simulink model "IEEE34_SPSload"  (R2021b)
settings: Solver=ode4  StartTime=0.0  StopTime=5  FixedStep=50e-6  RelTol=1e-3
PreLoadFcn:
  | pGain = 0.05; % Gain of random perturbation (pu)
  | pGainAP = 0.01; % Gain of sinusoidal active power variation (pu)
  | pGainRP = 0.01; % Gain of sinusoidal reactive power variation (pu)
  | pFreqAP = 0.03; % Frequency of sinusoidal active power variation (Hz)
  | pFreqRP = 0.03; % Frequency of sinusoidal reactive power variation (Hz)
  | 
  | init_IEEE34nodetestfeeder;
InitFcn:
  | pGain = 0.05; % Gain of random perturbation (pu)
  | pGainAP = 0.01; % Gain of sinusoidal active power variation (pu)
  | pGainRP = 0.01; % Gain of sinusoidal reactive power variation (pu)
  | pFreqAP = 0.03; % Frequency of sinusoidal active power variation (Hz)
  | pFreqRP = 0.03; % Frequency of sinusoidal reactive power variation (Hz)
  | 
  | init_IEEE34nodetestfeeder;
values from neighbouring files (symbols this model uses):
  fNom = f    (= 60)    [init_IEEE34nodetestfeeder.m]
  loadcoeff = 1.0    (= 1)    [init_IEEE34nodetestfeeder.m]
  Ts = 50e-6    (= 5e-05)    [init_IEEE34nodetestfeeder.m]
  vNomMV = VsubL    (= 24900)    [init_IEEE34nodetestfeeder.m]
  VsubL = 24.9e3    (= 24900)    [init_IEEE34nodetestfeeder.m]
  VxfmL = 4.16e3    (= 4160)    [init_IEEE34nodetestfeeder.m]
undefined symbols (not defined in the file or in its folder): Ac, Bc, Cc, Dc, find_system, j
libraries: spsSeriesRLCBranchLib x418, spsGroundLib x242, simulink_extras x176, spsVoltageMeasurementLib x106, spsRMSLib x96, spsControlledCurrentSourceLib x94, spsThreePhaseVIMeasurementLib x37, spsMutualInductanceLib x24, spsCurrentMeasurementLib x12, spsOnDelayLib x12, spsLinearTransformerLib x6, spsControlledVoltageSourceLib x6
(part 14 of 33)

== system IEEE34_SPSload/SM_IEEE34/DL_844-1/Load B2/model ==
  v : Inport
  PQ : Inport  Port=2
  Break Alg. Loop : Subsystem
  Complex to Magnitude-Angle : ComplexToMagnitudeAngle
  Complex to Real-Imag1 : ComplexToRealImag
  Constant : Constant
  Demux : Demux  Outputs=2
      settings: DisplayOption=none
  Divide : Product  Inputs=**
  IC1 : InitialCondition
  IC2 : InitialCondition
  Magnitude-Angle to Complex : MagnitudeAngleToComplex
  PLL : Subsystem  mask{freq=fnom}
      mask prompts: freq "Initial frequency (Hz)"
  Positive Sequence current : Subsystem
  RMS1 : spsRMSLib/RMS  TrueRMS=on  Freq=fnom  RMSInit=1  Ts=0
  Real-Imag to Complex : RealImagToComplex
  Real-Imag to Complex1 : RealImagToComplex
  Sum : Sum
  Trigonometric Function1 : Trigonometry
  V> pu : Gain  Gain=1/Vbase/sqrt(3)  SaturateOnIntegerOverflow=on  OutDataTypeStr=Inherit: Same as input  ParamDataTypeStr=Inherit: Same as input
  V> pu1 : Gain  Gain=sqrt(2)  SaturateOnIntegerOverflow=on  OutDataTypeStr=Inherit: Same as input  ParamDataTypeStr=Inherit: Same as input
  i : Outport  VectorParamsAs1DForOutWhenUnconnected=off
  m : Outport  Port=2  VectorParamsAs1DForOutWhenUnconnected=off
  wires:
  V> pu/1 -> PLL/1(v (pu)), V> pu1/1
  Real-Imag to Complex/1 -> Positive Sequence current/1(V1(pu))
  Positive Sequence current/1(I1(A)) -> Break Alg. Loop/1(In)
  PQ/1 -> Demux/1
  Demux/1 -> Real-Imag to Complex1/1
  Demux/2 -> Real-Imag to Complex1/2
  Real-Imag to Complex1/1 -> Positive Sequence current/2(S_ext)
  Positive Sequence current/2(VPQ) -> m/1
  v/1 -> IC2/1
  Complex to Real-Imag1/1 -> Real-Imag to Complex/1
  Complex to Real-Imag1/2 -> Real-Imag to Complex/2
  Magnitude-Angle to Complex/1 -> Complex to Real-Imag1/1
  Constant/1 -> PLL/2(freq (pu))
  PLL/1(alpha (rad)) -> Magnitude-Angle to Complex/2
  Complex to Magnitude-Angle/2 -> Sum/2
  PLL/2(wt) -> Sum/1
  Sum/1 -> Trigonometric Function1/1
  Trigonometric Function1/1 -> Divide/2
  Complex to Magnitude-Angle/1 -> Divide/1
  Divide/1 -> i/1
  Break Alg. Loop/1(Out) -> Complex to Magnitude-Angle/1
  RMS1/1 -> IC1/1
  IC1/1 -> Magnitude-Angle to Complex/1
  V> pu1/1 -> RMS1/1
  IC2/1 -> V> pu/1

== system IEEE34_SPSload/SM_IEEE34/DL_844-846/Load B/Measurement list ==
  In1 : Inport
  Bus Creator1 : BusCreator  Inputs=3
  Demux : Demux  Outputs=[1,1,1]
  Out1 : Outport  VectorParamsAs1DForOutWhenUnconnected=off
  wires:
  Demux/3 -> Bus Creator1/3  "Reactive power Q (var)"
  Demux/1 -> Bus Creator1/1  "Positive-sequence voltage V (pu)"
  Demux/2 -> Bus Creator1/2  "Active power P (W)"
  Bus Creator1/1 -> Out1/1
  In1/1 -> Demux/1

== system IEEE34_SPSload/SM_IEEE34/DL_844-846/Load B/model ==
  v : Inport
  PQ : Inport  Port=2
  Break Alg. Loop : Subsystem
  Complex to Magnitude-Angle : ComplexToMagnitudeAngle
  Complex to Real-Imag1 : ComplexToRealImag
  Constant : Constant
  Demux : Demux  Outputs=2
      settings: DisplayOption=none
  Divide : Product  Inputs=**
  IC1 : InitialCondition
  IC2 : InitialCondition
  Magnitude-Angle to Complex : MagnitudeAngleToComplex
  PLL : Subsystem  mask{freq=fnom}
      mask prompts: freq "Initial frequency (Hz)"
  Positive Sequence current : Subsystem
  RMS1 : spsRMSLib/RMS  TrueRMS=on  Freq=fnom  RMSInit=1  Ts=0
  Real-Imag to Complex : RealImagToComplex
  Real-Imag to Complex1 : RealImagToComplex
  Sum : Sum
  Trigonometric Function1 : Trigonometry
  V> pu : Gain  Gain=1/Vbase/sqrt(3)  SaturateOnIntegerOverflow=on  OutDataTypeStr=Inherit: Same as input  ParamDataTypeStr=Inherit: Same as input
  V> pu1 : Gain  Gain=sqrt(2)  SaturateOnIntegerOverflow=on  OutDataTypeStr=Inherit: Same as input  ParamDataTypeStr=Inherit: Same as input
  i : Outport  VectorParamsAs1DForOutWhenUnconnected=off
  m : Outport  Port=2  VectorParamsAs1DForOutWhenUnconnected=off
  wires:
  V> pu/1 -> PLL/1(v (pu)), V> pu1/1
  Real-Imag to Complex/1 -> Positive Sequence current/1(V1(pu))
  Positive Sequence current/1(I1(A)) -> Break Alg. Loop/1(In)
  PQ/1 -> Demux/1
  Demux/1 -> Real-Imag to Complex1/1
  Demux/2 -> Real-Imag to Complex1/2
  Real-Imag to Complex1/1 -> Positive Sequence current/2(S_ext)
  Positive Sequence current/2(VPQ) -> m/1
  v/1 -> IC2/1
  Complex to Real-Imag1/1 -> Real-Imag to Complex/1
  Complex to Real-Imag1/2 -> Real-Imag to Complex/2
  Magnitude-Angle to Complex/1 -> Complex to Real-Imag1/1
  Constant/1 -> PLL/2(freq (pu))
  PLL/1(alpha (rad)) -> Magnitude-Angle to Complex/2
  Complex to Magnitude-Angle/2 -> Sum/2
  PLL/2(wt) -> Sum/1
  Sum/1 -> Trigonometric Function1/1
  Trigonometric Function1/1 -> Divide/2
  Complex to Magnitude-Angle/1 -> Divide/1
  Divide/1 -> i/1
  Break Alg. Loop/1(Out) -> Complex to Magnitude-Angle/1
  RMS1/1 -> IC1/1
  IC1/1 -> Magnitude-Angle to Complex/1
  V> pu1/1 -> RMS1/1
  IC2/1 -> V> pu/1

== system IEEE34_SPSload/SM_IEEE34/DL_844-846/Load B1/Measurement list ==
  In1 : Inport
  Bus Creator1 : BusCreator  Inputs=3
  Demux : Demux  Outputs=[1,1,1]
  Out1 : Outport  VectorParamsAs1DForOutWhenUnconnected=off
  wires:
  Demux/3 -> Bus Creator1/3  "Reactive power Q (var)"
  Demux/1 -> Bus Creator1/1  "Positive-sequence voltage V (pu)"
  Demux/2 -> Bus Creator1/2  "Active power P (W)"
  Bus Creator1/1 -> Out1/1
  In1/1 -> Demux/1

== system IEEE34_SPSload/SM_IEEE34/DL_844-846/Load B1/model ==
  v : Inport
  PQ : Inport  Port=2
  Break Alg. Loop : Subsystem
  Complex to Magnitude-Angle : ComplexToMagnitudeAngle
  Complex to Real-Imag1 : ComplexToRealImag
  Constant : Constant
  Demux : Demux  Outputs=2
      settings: DisplayOption=none
  Divide : Product  Inputs=**
  IC1 : InitialCondition
  IC2 : InitialCondition
  Magnitude-Angle to Complex : MagnitudeAngleToComplex
  PLL : Subsystem  mask{freq=fnom}
      mask prompts: freq "Initial frequency (Hz)"
  Positive Sequence current : Subsystem
  RMS1 : spsRMSLib/RMS  TrueRMS=on  Freq=fnom  RMSInit=1  Ts=0
  Real-Imag to Complex : RealImagToComplex
  Real-Imag to Complex1 : RealImagToComplex
  Sum : Sum
  Trigonometric Function1 : Trigonometry
  V> pu : Gain  Gain=1/Vbase/sqrt(3)  SaturateOnIntegerOverflow=on  OutDataTypeStr=Inherit: Same as input  ParamDataTypeStr=Inherit: Same as input
  V> pu1 : Gain  Gain=sqrt(2)  SaturateOnIntegerOverflow=on  OutDataTypeStr=Inherit: Same as input  ParamDataTypeStr=Inherit: Same as input
  i : Outport  VectorParamsAs1DForOutWhenUnconnected=off
  m : Outport  Port=2  VectorParamsAs1DForOutWhenUnconnected=off
  wires:
  V> pu/1 -> PLL/1(v (pu)), V> pu1/1
  Real-Imag to Complex/1 -> Positive Sequence current/1(V1(pu))
  Positive Sequence current/1(I1(A)) -> Break Alg. Loop/1(In)
  PQ/1 -> Demux/1
  Demux/1 -> Real-Imag to Complex1/1
  Demux/2 -> Real-Imag to Complex1/2
  Real-Imag to Complex1/1 -> Positive Sequence current/2(S_ext)
  Positive Sequence current/2(VPQ) -> m/1
  v/1 -> IC2/1
  Complex to Real-Imag1/1 -> Real-Imag to Complex/1
  Complex to Real-Imag1/2 -> Real-Imag to Complex/2
  Magnitude-Angle to Complex/1 -> Complex to Real-Imag1/1
  Constant/1 -> PLL/2(freq (pu))
  PLL/1(alpha (rad)) -> Magnitude-Angle to Complex/2
  Complex to Magnitude-Angle/2 -> Sum/2
  PLL/2(wt) -> Sum/1
  Sum/1 -> Trigonometric Function1/1
  Trigonometric Function1/1 -> Divide/2
  Complex to Magnitude-Angle/1 -> Divide/1
  Divide/1 -> i/1
  Break Alg. Loop/1(Out) -> Complex to Magnitude-Angle/1
  RMS1/1 -> IC1/1
  IC1/1 -> Magnitude-Angle to Complex/1
  V> pu1/1 -> RMS1/1
  IC2/1 -> V> pu/1

== system IEEE34_SPSload/SM_IEEE34/DL_844-846/Load B2/Measurement list ==
  In1 : Inport
  Bus Creator1 : BusCreator  Inputs=3
  Demux : Demux  Outputs=[1,1,1]
  Out1 : Outport  VectorParamsAs1DForOutWhenUnconnected=off
  wires:
  In1/1 -> Demux/1
  Bus Creator1/1 -> Out1/1
  Demux/2 -> Bus Creator1/2  "Active power P (W)"
  Demux/1 -> Bus Creator1/1  "Positive-sequence voltage V (pu)"
  Demux/3 -> Bus Creator1/3  "Reactive power Q (var)"

== system IEEE34_SPSload/SM_IEEE34/DL_844-846/Load B2/model ==
  v : Inport
  PQ : Inport  Port=2
  Break Alg. Loop : Subsystem
  Complex to Magnitude-Angle : ComplexToMagnitudeAngle
  Complex to Real-Imag1 : ComplexToRealImag
  Constant : Constant
  Demux : Demux  Outputs=2
      settings: DisplayOption=none
  Divide : Product  Inputs=**
  IC1 : InitialCondition
  IC2 : InitialCondition
  Magnitude-Angle to Complex : MagnitudeAngleToComplex
  PLL : Subsystem  mask{freq=fnom}
      mask prompts: freq "Initial frequency (Hz)"
  Positive Sequence current : Subsystem
  RMS1 : spsRMSLib/RMS  TrueRMS=on  Freq=fnom  RMSInit=1  Ts=0
  Real-Imag to Complex : RealImagToComplex
  Real-Imag to Complex1 : RealImagToComplex
  Sum : Sum
  Trigonometric Function1 : Trigonometry
  V> pu : Gain  Gain=1/Vbase/sqrt(3)  SaturateOnIntegerOverflow=on  OutDataTypeStr=Inherit: Same as input  ParamDataTypeStr=Inherit: Same as input
  V> pu1 : Gain  Gain=sqrt(2)  SaturateOnIntegerOverflow=on  OutDataTypeStr=Inherit: Same as input  ParamDataTypeStr=Inherit: Same as input
  i : Outport  VectorParamsAs1DForOutWhenUnconnected=off
  m : Outport  Port=2  VectorParamsAs1DForOutWhenUnconnected=off
  wires:
  IC2/1 -> V> pu/1
  V> pu1/1 -> RMS1/1
  IC1/1 -> Magnitude-Angle to Complex/1
  RMS1/1 -> IC1/1
  Break Alg. Loop/1(Out) -> Complex to Magnitude-Angle/1
  Divide/1 -> i/1
  Complex to Magnitude-Angle/1 -> Divide/1
  Trigonometric Function1/1 -> Divide/2
  Sum/1 -> Trigonometric Function1/1
  PLL/2(wt) -> Sum/1
  Complex to Magnitude-Angle/2 -> Sum/2
  PLL/1(alpha (rad)) -> Magnitude-Angle to Complex/2
  Constant/1 -> PLL/2(freq (pu))
  Magnitude-Angle to Complex/1 -> Complex to Real-Imag1/1
  Complex to Real-Imag1/2 -> Real-Imag to Complex/2
  Complex to Real-Imag1/1 -> Real-Imag to Complex/1
  v/1 -> IC2/1
  Positive Sequence current/2(VPQ) -> m/1
  Real-Imag to Complex1/1 -> Positive Sequence current/2(S_ext)
  Demux/2 -> Real-Imag to Complex1/2
  Demux/1 -> Real-Imag to Complex1/1
  PQ/1 -> Demux/1
  Positive Sequence current/1(I1(A)) -> Break Alg. Loop/1(In)
  Real-Imag to Complex/1 -> Positive Sequence current/1(V1(pu))
  V> pu/1 -> V> pu1/1, PLL/1(v (pu))

== system IEEE34_SPSload/SM_IEEE34/DL_846-1/Load B/Measurement list ==
  In1 : Inport
  Bus Creator1 : BusCreator  Inputs=3
  Demux : Demux  Outputs=[1,1,1]
  Out1 : Outport  VectorParamsAs1DForOutWhenUnconnected=off
  wires:
  In1/1 -> Demux/1
  Bus Creator1/1 -> Out1/1
  Demux/2 -> Bus Creator1/2  "Active power P (W)"
  Demux/1 -> Bus Creator1/1  "Positive-sequence voltage V (pu)"
  Demux/3 -> Bus Creator1/3  "Reactive power Q (var)"

== system IEEE34_SPSload/SM_IEEE34/DL_846-1/Load B/model ==
  v : Inport
  PQ : Inport  Port=2
  Break Alg. Loop : Subsystem
  Complex to Magnitude-Angle : ComplexToMagnitudeAngle
  Complex to Real-Imag1 : ComplexToRealImag
  Constant : Constant
  Demux : Demux  Outputs=2
      settings: DisplayOption=none
  Divide : Product  Inputs=**
  IC1 : InitialCondition
  IC2 : InitialCondition
  Magnitude-Angle to Complex : MagnitudeAngleToComplex
  PLL : Subsystem  mask{freq=fnom}
      mask prompts: freq "Initial frequency (Hz)"
  Positive Sequence current : Subsystem
  RMS1 : spsRMSLib/RMS  TrueRMS=on  Freq=fnom  RMSInit=1  Ts=0
  Real-Imag to Complex : RealImagToComplex
  Real-Imag to Complex1 : RealImagToComplex
  Sum : Sum
  Trigonometric Function1 : Trigonometry
  V> pu : Gain  Gain=1/Vbase/sqrt(3)  SaturateOnIntegerOverflow=on  OutDataTypeStr=Inherit: Same as input  ParamDataTypeStr=Inherit: Same as input
  V> pu1 : Gain  Gain=sqrt(2)  SaturateOnIntegerOverflow=on  OutDataTypeStr=Inherit: Same as input  ParamDataTypeStr=Inherit: Same as input
  i : Outport  VectorParamsAs1DForOutWhenUnconnected=off
  m : Outport  Port=2  VectorParamsAs1DForOutWhenUnconnected=off
  wires:
  IC2/1 -> V> pu/1
  V> pu1/1 -> RMS1/1
  IC1/1 -> Magnitude-Angle to Complex/1
  RMS1/1 -> IC1/1
  Break Alg. Loop/1(Out) -> Complex to Magnitude-Angle/1
  Divide/1 -> i/1
  Complex to Magnitude-Angle/1 -> Divide/1
  Trigonometric Function1/1 -> Divide/2
  Sum/1 -> Trigonometric Function1/1
  PLL/2(wt) -> Sum/1
  Complex to Magnitude-Angle/2 -> Sum/2
  PLL/1(alpha (rad)) -> Magnitude-Angle to Complex/2
  Constant/1 -> PLL/2(freq (pu))
  Magnitude-Angle to Complex/1 -> Complex to Real-Imag1/1
  Complex to Real-Imag1/2 -> Real-Imag to Complex/2
  Complex to Real-Imag1/1 -> Real-Imag to Complex/1
  v/1 -> IC2/1
  Positive Sequence current/2(VPQ) -> m/1
  Real-Imag to Complex1/1 -> Positive Sequence current/2(S_ext)
  Demux/2 -> Real-Imag to Complex1/2
  Demux/1 -> Real-Imag to Complex1/1
  PQ/1 -> Demux/1
  Positive Sequence current/1(I1(A)) -> Break Alg. Loop/1(In)
  Real-Imag to Complex/1 -> Positive Sequence current/1(V1(pu))
  V> pu/1 -> V> pu1/1, PLL/1(v (pu))

== system IEEE34_SPSload/SM_IEEE34/DL_846-848/Load B/Measurement list ==
  In1 : Inport
  Bus Creator1 : BusCreator  Inputs=3
  Demux : Demux  Outputs=[1,1,1]
  Out1 : Outport  VectorParamsAs1DForOutWhenUnconnected=off
  wires:
  Demux/3 -> Bus Creator1/3  "Reactive power Q (var)"
  Demux/1 -> Bus Creator1/1  "Positive-sequence voltage V (pu)"
  Demux/2 -> Bus Creator1/2  "Active power P (W)"
  Bus Creator1/1 -> Out1/1
  In1/1 -> Demux/1

== system IEEE34_SPSload/SM_IEEE34/DL_846-848/Load B/model ==
  v : Inport
  PQ : Inport  Port=2
  Break Alg. Loop : Subsystem
  Complex to Magnitude-Angle : ComplexToMagnitudeAngle
  Complex to Real-Imag1 : ComplexToRealImag
  Constant : Constant
  Demux : Demux  Outputs=2
      settings: DisplayOption=none
  Divide : Product  Inputs=**
  IC1 : InitialCondition
  IC2 : InitialCondition
  Magnitude-Angle to Complex : MagnitudeAngleToComplex
  PLL : Subsystem  mask{freq=fnom}
      mask prompts: freq "Initial frequency (Hz)"
  Positive Sequence current : Subsystem
  RMS1 : spsRMSLib/RMS  TrueRMS=on  Freq=fnom  RMSInit=1  Ts=0
  Real-Imag to Complex : RealImagToComplex
  Real-Imag to Complex1 : RealImagToComplex
  Sum : Sum
  Trigonometric Function1 : Trigonometry
  V> pu : Gain  Gain=1/Vbase/sqrt(3)  SaturateOnIntegerOverflow=on  OutDataTypeStr=Inherit: Same as input  ParamDataTypeStr=Inherit: Same as input
  V> pu1 : Gain  Gain=sqrt(2)  SaturateOnIntegerOverflow=on  OutDataTypeStr=Inherit: Same as input  ParamDataTypeStr=Inherit: Same as input
  i : Outport  VectorParamsAs1DForOutWhenUnconnected=off
  m : Outport  Port=2  VectorParamsAs1DForOutWhenUnconnected=off
  wires:
  V> pu/1 -> PLL/1(v (pu)), V> pu1/1
  Real-Imag to Complex/1 -> Positive Sequence current/1(V1(pu))
  Positive Sequence current/1(I1(A)) -> Break Alg. Loop/1(In)
  PQ/1 -> Demux/1
  Demux/1 -> Real-Imag to Complex1/1
  Demux/2 -> Real-Imag to Complex1/2
  Real-Imag to Complex1/1 -> Positive Sequence current/2(S_ext)
  Positive Sequence current/2(VPQ) -> m/1
  v/1 -> IC2/1
  Complex to Real-Imag1/1 -> Real-Imag to Complex/1
  Complex to Real-Imag1/2 -> Real-Imag to Complex/2
  Magnitude-Angle to Complex/1 -> Complex to Real-Imag1/1
  Constant/1 -> PLL/2(freq (pu))
  PLL/1(alpha (rad)) -> Magnitude-Angle to Complex/2
  Complex to Magnitude-Angle/2 -> Sum/2
  PLL/2(wt) -> Sum/1
  Sum/1 -> Trigonometric Function1/1
  Trigonometric Function1/1 -> Divide/2
  Complex to Magnitude-Angle/1 -> Divide/1
  Divide/1 -> i/1
  Break Alg. Loop/1(Out) -> Complex to Magnitude-Angle/1
  RMS1/1 -> IC1/1
  IC1/1 -> Magnitude-Angle to Complex/1
  V> pu1/1 -> RMS1/1
  IC2/1 -> V> pu/1

== system IEEE34_SPSload/SM_IEEE34/DL_854-1/Load B/Measurement list ==
  In1 : Inport
  Bus Creator1 : BusCreator  Inputs=3
  Demux : Demux  Outputs=[1,1,1]
  Out1 : Outport  VectorParamsAs1DForOutWhenUnconnected=off
  wires:
  In1/1 -> Demux/1
  Bus Creator1/1 -> Out1/1
  Demux/2 -> Bus Creator1/2  "Active power P (W)"
  Demux/1 -> Bus Creator1/1  "Positive-sequence voltage V (pu)"
  Demux/3 -> Bus Creator1/3  "Reactive power Q (var)"

== system IEEE34_SPSload/SM_IEEE34/DL_854-1/Load B/model ==
  v : Inport
  PQ : Inport  Port=2
  Break Alg. Loop : Subsystem
  Complex to Magnitude-Angle : ComplexToMagnitudeAngle
  Complex to Real-Imag1 : ComplexToRealImag
  Constant : Constant
  Demux : Demux  Outputs=2
      settings: DisplayOption=none
  Divide : Product  Inputs=**
  IC1 : InitialCondition
  IC2 : InitialCondition
  Magnitude-Angle to Complex : MagnitudeAngleToComplex
  PLL : Subsystem  mask{freq=fnom}
      mask prompts: freq "Initial frequency (Hz)"
  Positive Sequence current : Subsystem
  RMS1 : spsRMSLib/RMS  TrueRMS=on  Freq=fnom  RMSInit=1  Ts=0
  Real-Imag to Complex : RealImagToComplex
  Real-Imag to Complex1 : RealImagToComplex
  Sum : Sum
  Trigonometric Function1 : Trigonometry
  V> pu : Gain  Gain=1/Vbase/sqrt(3)  SaturateOnIntegerOverflow=on  OutDataTypeStr=Inherit: Same as input  ParamDataTypeStr=Inherit: Same as input
  V> pu1 : Gain  Gain=sqrt(2)  SaturateOnIntegerOverflow=on  OutDataTypeStr=Inherit: Same as input  ParamDataTypeStr=Inherit: Same as input
  i : Outport  VectorParamsAs1DForOutWhenUnconnected=off
  m : Outport  Port=2  VectorParamsAs1DForOutWhenUnconnected=off
  wires:
  IC2/1 -> V> pu/1
  V> pu1/1 -> RMS1/1
  IC1/1 -> Magnitude-Angle to Complex/1
  RMS1/1 -> IC1/1
  Break Alg. Loop/1(Out) -> Complex to Magnitude-Angle/1
  Divide/1 -> i/1
  Complex to Magnitude-Angle/1 -> Divide/1
  Trigonometric Function1/1 -> Divide/2
  Sum/1 -> Trigonometric Function1/1
  PLL/2(wt) -> Sum/1
  Complex to Magnitude-Angle/2 -> Sum/2
  PLL/1(alpha (rad)) -> Magnitude-Angle to Complex/2
  Constant/1 -> PLL/2(freq (pu))
  Magnitude-Angle to Complex/1 -> Complex to Real-Imag1/1
  Complex to Real-Imag1/2 -> Real-Imag to Complex/2
  Complex to Real-Imag1/1 -> Real-Imag to Complex/1
  v/1 -> IC2/1
  Positive Sequence current/2(VPQ) -> m/1
  Real-Imag to Complex1/1 -> Positive Sequence current/2(S_ext)
  Demux/2 -> Real-Imag to Complex1/2
  Demux/1 -> Real-Imag to Complex1/1
  PQ/1 -> Demux/1
  Positive Sequence current/1(I1(A)) -> Break Alg. Loop/1(In)
  Real-Imag to Complex/1 -> Positive Sequence current/1(V1(pu))
  V> pu/1 -> V> pu1/1, PLL/1(v (pu))

== system IEEE34_SPSload/SM_IEEE34/DL_854-856/Load B/Measurement list ==
  In1 : Inport
  Bus Creator1 : BusCreator  Inputs=3
  Demux : Demux  Outputs=[1,1,1]
  Out1 : Outport  VectorParamsAs1DForOutWhenUnconnected=off
  wires:
  Demux/3 -> Bus Creator1/3  "Reactive power Q (var)"
  Demux/1 -> Bus Creator1/1  "Positive-sequence voltage V (pu)"
  Demux/2 -> Bus Creator1/2  "Active power P (W)"
  Bus Creator1/1 -> Out1/1
  In1/1 -> Demux/1

== system IEEE34_SPSload/SM_IEEE34/DL_854-856/Load B/model ==
  v : Inport
  PQ : Inport  Port=2
  Break Alg. Loop : Subsystem
  Complex to Magnitude-Angle : ComplexToMagnitudeAngle
  Complex to Real-Imag1 : ComplexToRealImag
  Constant : Constant
  Demux : Demux  Outputs=2
      settings: DisplayOption=none
  Divide : Product  Inputs=**
  IC1 : InitialCondition
  IC2 : InitialCondition
  Magnitude-Angle to Complex : MagnitudeAngleToComplex
  PLL : Subsystem  mask{freq=fnom}
      mask prompts: freq "Initial frequency (Hz)"
  Positive Sequence current : Subsystem
  RMS1 : spsRMSLib/RMS  TrueRMS=on  Freq=fnom  RMSInit=1  Ts=0
  Real-Imag to Complex : RealImagToComplex
  Real-Imag to Complex1 : RealImagToComplex
  Sum : Sum
  Trigonometric Function1 : Trigonometry
  V> pu : Gain  Gain=1/Vbase/sqrt(3)  SaturateOnIntegerOverflow=on  OutDataTypeStr=Inherit: Same as input  ParamDataTypeStr=Inherit: Same as input
  V> pu1 : Gain  Gain=sqrt(2)  SaturateOnIntegerOverflow=on  OutDataTypeStr=Inherit: Same as input  ParamDataTypeStr=Inherit: Same as input
  i : Outport  VectorParamsAs1DForOutWhenUnconnected=off
  m : Outport  Port=2  VectorParamsAs1DForOutWhenUnconnected=off
  wires:
  V> pu/1 -> PLL/1(v (pu)), V> pu1/1
  Real-Imag to Complex/1 -> Positive Sequence current/1(V1(pu))
  Positive Sequence current/1(I1(A)) -> Break Alg. Loop/1(In)
  PQ/1 -> Demux/1
  Demux/1 -> Real-Imag to Complex1/1
  Demux/2 -> Real-Imag to Complex1/2
  Real-Imag to Complex1/1 -> Positive Sequence current/2(S_ext)
  Positive Sequence current/2(VPQ) -> m/1
  v/1 -> IC2/1
  Complex to Real-Imag1/1 -> Real-Imag to Complex/1
  Complex to Real-Imag1/2 -> Real-Imag to Complex/2
  Magnitude-Angle to Complex/1 -> Complex to Real-Imag1/1
  Constant/1 -> PLL/2(freq (pu))
  PLL/1(alpha (rad)) -> Magnitude-Angle to Complex/2
  Complex to Magnitude-Angle/2 -> Sum/2
  PLL/2(wt) -> Sum/1
  Sum/1 -> Trigonometric Function1/1
  Trigonometric Function1/1 -> Divide/2
  Complex to Magnitude-Angle/1 -> Divide/1
  Divide/1 -> i/1
  Break Alg. Loop/1(Out) -> Complex to Magnitude-Angle/1
  RMS1/1 -> IC1/1
  IC1/1 -> Magnitude-Angle to Complex/1
  V> pu1/1 -> RMS1/1
  IC2/1 -> V> pu/1

== system IEEE34_SPSload/SM_IEEE34/DL_858-1/Load B/Measurement list ==
  In1 : Inport
  Bus Creator1 : BusCreator  Inputs=3
  Demux : Demux  Outputs=[1,1,1]
  Out1 : Outport  VectorParamsAs1DForOutWhenUnconnected=off
  wires:
  In1/1 -> Demux/1
  Bus Creator1/1 -> Out1/1
  Demux/2 -> Bus Creator1/2  "Active power P (W)"
  Demux/1 -> Bus Creator1/1  "Positive-sequence voltage V (pu)"
  Demux/3 -> Bus Creator1/3  "Reactive power Q (var)"

== system IEEE34_SPSload/SM_IEEE34/DL_858-1/Load B/model ==
  v : Inport
  PQ : Inport  Port=2
  Break Alg. Loop : Subsystem
  Complex to Magnitude-Angle : ComplexToMagnitudeAngle
  Complex to Real-Imag1 : ComplexToRealImag
  Constant : Constant
  Demux : Demux  Outputs=2
      settings: DisplayOption=none
  Divide : Product  Inputs=**
  IC1 : InitialCondition
  IC2 : InitialCondition
  Magnitude-Angle to Complex : MagnitudeAngleToComplex
  PLL : Subsystem  mask{freq=fnom}
      mask prompts: freq "Initial frequency (Hz)"
  Positive Sequence current : Subsystem
  RMS1 : spsRMSLib/RMS  TrueRMS=on  Freq=fnom  RMSInit=1  Ts=0
  Real-Imag to Complex : RealImagToComplex
  Real-Imag to Complex1 : RealImagToComplex
  Sum : Sum
  Trigonometric Function1 : Trigonometry
  V> pu : Gain  Gain=1/Vbase/sqrt(3)  SaturateOnIntegerOverflow=on  OutDataTypeStr=Inherit: Same as input  ParamDataTypeStr=Inherit: Same as input
  V> pu1 : Gain  Gain=sqrt(2)  SaturateOnIntegerOverflow=on  OutDataTypeStr=Inherit: Same as input  ParamDataTypeStr=Inherit: Same as input
  i : Outport  VectorParamsAs1DForOutWhenUnconnected=off
  m : Outport  Port=2  VectorParamsAs1DForOutWhenUnconnected=off
  wires:
  IC2/1 -> V> pu/1
  V> pu1/1 -> RMS1/1
  IC1/1 -> Magnitude-Angle to Complex/1
  RMS1/1 -> IC1/1
  Break Alg. Loop/1(Out) -> Complex to Magnitude-Angle/1
  Divide/1 -> i/1
  Complex to Magnitude-Angle/1 -> Divide/1
  Trigonometric Function1/1 -> Divide/2
  Sum/1 -> Trigonometric Function1/1
  PLL/2(wt) -> Sum/1
  Complex to Magnitude-Angle/2 -> Sum/2
  PLL/1(alpha (rad)) -> Magnitude-Angle to Complex/2
  Constant/1 -> PLL/2(freq (pu))
  Magnitude-Angle to Complex/1 -> Complex to Real-Imag1/1
  Complex to Real-Imag1/2 -> Real-Imag to Complex/2
  Complex to Real-Imag1/1 -> Real-Imag to Complex/1
  v/1 -> IC2/1
  Positive Sequence current/2(VPQ) -> m/1
  Real-Imag to Complex1/1 -> Positive Sequence current/2(S_ext)
  Demux/2 -> Real-Imag to Complex1/2
  Demux/1 -> Real-Imag to Complex1/1
  PQ/1 -> Demux/1
  Positive Sequence current/1(I1(A)) -> Break Alg. Loop/1(In)
  Real-Imag to Complex/1 -> Positive Sequence current/1(V1(pu))
  V> pu/1 -> V> pu1/1, PLL/1(v (pu))

== system IEEE34_SPSload/SM_IEEE34/DL_858-2/Load B/Measurement list ==
  In1 : Inport
  Bus Creator1 : BusCreator  Inputs=3
  Demux : Demux  Outputs=[1,1,1]
  Out1 : Outport  VectorParamsAs1DForOutWhenUnconnected=off
  wires:
  In1/1 -> Demux/1
  Bus Creator1/1 -> Out1/1
  Demux/2 -> Bus Creator1/2  "Active power P (W)"
  Demux/1 -> Bus Creator1/1  "Positive-sequence voltage V (pu)"
  Demux/3 -> Bus Creator1/3  "Reactive power Q (var)"

== system IEEE34_SPSload/SM_IEEE34/DL_858-2/Load B/model ==
  v : Inport
  PQ : Inport  Port=2
  Break Alg. Loop : Subsystem
  Complex to Magnitude-Angle : ComplexToMagnitudeAngle
  Complex to Real-Imag1 : ComplexToRealImag
  Constant : Constant
  Demux : Demux  Outputs=2
      settings: DisplayOption=none
  Divide : Product  Inputs=**
  IC1 : InitialCondition
  IC2 : InitialCondition
  Magnitude-Angle to Complex : MagnitudeAngleToComplex
  PLL : Subsystem  mask{freq=fnom}
      mask prompts: freq "Initial frequency (Hz)"
  Positive Sequence current : Subsystem
  RMS1 : spsRMSLib/RMS  TrueRMS=on  Freq=fnom  RMSInit=1  Ts=0
  Real-Imag to Complex : RealImagToComplex
  Real-Imag to Complex1 : RealImagToComplex
  Sum : Sum
  Trigonometric Function1 : Trigonometry
  V> pu : Gain  Gain=1/Vbase/sqrt(3)  SaturateOnIntegerOverflow=on  OutDataTypeStr=Inherit: Same as input  ParamDataTypeStr=Inherit: Same as input
  V> pu1 : Gain  Gain=sqrt(2)  SaturateOnIntegerOverflow=on  OutDataTypeStr=Inherit: Same as input  ParamDataTypeStr=Inherit: Same as input
  i : Outport  VectorParamsAs1DForOutWhenUnconnected=off
  m : Outport  Port=2  VectorParamsAs1DForOutWhenUnconnected=off
  wires:
  IC2/1 -> V> pu/1
  V> pu1/1 -> RMS1/1
  IC1/1 -> Magnitude-Angle to Complex/1
  RMS1/1 -> IC1/1
  Break Alg. Loop/1(Out) -> Complex to Magnitude-Angle/1
  Divide/1 -> i/1
  Complex to Magnitude-Angle/1 -> Divide/1
  Trigonometric Function1/1 -> Divide/2
  Sum/1 -> Trigonometric Function1/1
  PLL/2(wt) -> Sum/1
  Complex to Magnitude-Angle/2 -> Sum/2
  PLL/1(alpha (rad)) -> Magnitude-Angle to Complex/2
  Constant/1 -> PLL/2(freq (pu))
  Magnitude-Angle to Complex/1 -> Complex to Real-Imag1/1
  Complex to Real-Imag1/2 -> Real-Imag to Complex/2
  Complex to Real-Imag1/1 -> Real-Imag to Complex/1
  v/1 -> IC2/1
  Positive Sequence current/2(VPQ) -> m/1
  Real-Imag to Complex1/1 -> Positive Sequence current/2(S_ext)
  Demux/2 -> Real-Imag to Complex1/2
  Demux/1 -> Real-Imag to Complex1/1
  PQ/1 -> Demux/1
  Positive Sequence current/1(I1(A)) -> Break Alg. Loop/1(In)
  Real-Imag to Complex/1 -> Positive Sequence current/1(V1(pu))
  V> pu/1 -> V> pu1/1, PLL/1(v (pu))

== system IEEE34_SPSload/SM_IEEE34/DL_858-2/Load B1/Measurement list ==
  In1 : Inport
  Bus Creator1 : BusCreator  Inputs=3
  Demux : Demux  Outputs=[1,1,1]
  Out1 : Outport  VectorParamsAs1DForOutWhenUnconnected=off
  wires:
  In1/1 -> Demux/1
  Bus Creator1/1 -> Out1/1
  Demux/2 -> Bus Creator1/2  "Active power P (W)"
  Demux/1 -> Bus Creator1/1  "Positive-sequence voltage V (pu)"
  Demux/3 -> Bus Creator1/3  "Reactive power Q (var)"

== system IEEE34_SPSload/SM_IEEE34/DL_858-2/Load B1/model ==
  v : Inport
  PQ : Inport  Port=2
  Break Alg. Loop : Subsystem
  Complex to Magnitude-Angle : ComplexToMagnitudeAngle
  Complex to Real-Imag1 : ComplexToRealImag
  Constant : Constant
  Demux : Demux  Outputs=2
      settings: DisplayOption=none
  Divide : Product  Inputs=**
  IC1 : InitialCondition
  IC2 : InitialCondition
  Magnitude-Angle to Complex : MagnitudeAngleToComplex
  PLL : Subsystem  mask{freq=fnom}
      mask prompts: freq "Initial frequency (Hz)"
  Positive Sequence current : Subsystem
  RMS1 : spsRMSLib/RMS  TrueRMS=on  Freq=fnom  RMSInit=1  Ts=0
  Real-Imag to Complex : RealImagToComplex
  Real-Imag to Complex1 : RealImagToComplex
  Sum : Sum
  Trigonometric Function1 : Trigonometry
  V> pu : Gain  Gain=1/Vbase/sqrt(3)  SaturateOnIntegerOverflow=on  OutDataTypeStr=Inherit: Same as input  ParamDataTypeStr=Inherit: Same as input
  V> pu1 : Gain  Gain=sqrt(2)  SaturateOnIntegerOverflow=on  OutDataTypeStr=Inherit: Same as input  ParamDataTypeStr=Inherit: Same as input
  i : Outport  VectorParamsAs1DForOutWhenUnconnected=off
  m : Outport  Port=2  VectorParamsAs1DForOutWhenUnconnected=off
  wires:
  IC2/1 -> V> pu/1
  V> pu1/1 -> RMS1/1
  IC1/1 -> Magnitude-Angle to Complex/1
  RMS1/1 -> IC1/1
  Break Alg. Loop/1(Out) -> Complex to Magnitude-Angle/1
  Divide/1 -> i/1
  Complex to Magnitude-Angle/1 -> Divide/1
  Trigonometric Function1/1 -> Divide/2
  Sum/1 -> Trigonometric Function1/1
  PLL/2(wt) -> Sum/1
  Complex to Magnitude-Angle/2 -> Sum/2
  PLL/1(alpha (rad)) -> Magnitude-Angle to Complex/2
  Constant/1 -> PLL/2(freq (pu))
  Magnitude-Angle to Complex/1 -> Complex to Real-Imag1/1
  Complex to Real-Imag1/2 -> Real-Imag to Complex/2
  Complex to Real-Imag1/1 -> Real-Imag to Complex/1
  v/1 -> IC2/1
  Positive Sequence current/2(VPQ) -> m/1
  Real-Imag to Complex1/1 -> Positive Sequence current/2(S_ext)
  Demux/2 -> Real-Imag to Complex1/2
  Demux/1 -> Real-Imag to Complex1/1
  PQ/1 -> Demux/1
  Positive Sequence current/1(I1(A)) -> Break Alg. Loop/1(In)
  Real-Imag to Complex/1 -> Positive Sequence current/1(V1(pu))
  V> pu/1 -> V> pu1/1, PLL/1(v (pu))

== system IEEE34_SPSload/SM_IEEE34/DL_858-2/Load B2/Measurement list ==
  In1 : Inport
  Bus Creator1 : BusCreator  Inputs=3
  Demux : Demux  Outputs=[1,1,1]
  Out1 : Outport  VectorParamsAs1DForOutWhenUnconnected=off
  wires:
  In1/1 -> Demux/1
  Bus Creator1/1 -> Out1/1
  Demux/2 -> Bus Creator1/2  "Active power P (W)"
  Demux/1 -> Bus Creator1/1  "Positive-sequence voltage V (pu)"
  Demux/3 -> Bus Creator1/3  "Reactive power Q (var)"

== system IEEE34_SPSload/SM_IEEE34/DL_858-2/Load B2/model ==
  v : Inport
  PQ : Inport  Port=2
  Break Alg. Loop : Subsystem
  Complex to Magnitude-Angle : ComplexToMagnitudeAngle
  Complex to Real-Imag1 : ComplexToRealImag
  Constant : Constant
  Demux : Demux  Outputs=2
      settings: DisplayOption=none
  Divide : Product  Inputs=**
  IC1 : InitialCondition
  IC2 : InitialCondition
  Magnitude-Angle to Complex : MagnitudeAngleToComplex
  PLL : Subsystem  mask{freq=fnom}
      mask prompts: freq "Initial frequency (Hz)"
  Positive Sequence current : Subsystem
  RMS1 : spsRMSLib/RMS  TrueRMS=on  Freq=fnom  RMSInit=1  Ts=0
  Real-Imag to Complex : RealImagToComplex
  Real-Imag to Complex1 : RealImagToComplex
  Sum : Sum
  Trigonometric Function1 : Trigonometry
  V> pu : Gain  Gain=1/Vbase/sqrt(3)  SaturateOnIntegerOverflow=on  OutDataTypeStr=Inherit: Same as input  ParamDataTypeStr=Inherit: Same as input
  V> pu1 : Gain  Gain=sqrt(2)  SaturateOnIntegerOverflow=on  OutDataTypeStr=Inherit: Same as input  ParamDataTypeStr=Inherit: Same as input
  i : Outport  VectorParamsAs1DForOutWhenUnconnected=off
  m : Outport  Port=2  VectorParamsAs1DForOutWhenUnconnected=off
  wires:
  IC2/1 -> V> pu/1
  V> pu1/1 -> RMS1/1
  IC1/1 -> Magnitude-Angle to Complex/1
  RMS1/1 -> IC1/1
  Break Alg. Loop/1(Out) -> Complex to Magnitude-Angle/1
  Divide/1 -> i/1
  Complex to Magnitude-Angle/1 -> Divide/1
  Trigonometric Function1/1 -> Divide/2
  Sum/1 -> Trigonometric Function1/1
  PLL/2(wt) -> Sum/1
  Complex to Magnitude-Angle/2 -> Sum/2
  PLL/1(alpha (rad)) -> Magnitude-Angle to Complex/2
  Constant/1 -> PLL/2(freq (pu))
  Magnitude-Angle to Complex/1 -> Complex to Real-Imag1/1
  Complex to Real-Imag1/2 -> Real-Imag to Complex/2
  Complex to Real-Imag1/1 -> Real-Imag to Complex/1
  v/1 -> IC2/1
  Positive Sequence current/2(VPQ) -> m/1
  Real-Imag to Complex1/1 -> Positive Sequence current/2(S_ext)
  Demux/2 -> Real-Imag to Complex1/2
  Demux/1 -> Real-Imag to Complex1/1
  PQ/1 -> Demux/1
  Positive Sequence current/1(I1(A)) -> Break Alg. Loop/1(In)
  Real-Imag to Complex/1 -> Positive Sequence current/1(V1(pu))
  V> pu/1 -> V> pu1/1, PLL/1(v (pu))

== system IEEE34_SPSload/SM_IEEE34/DL_858-834/Load B/Measurement list ==
  In1 : Inport
  Bus Creator1 : BusCreator  Inputs=3
  Demux : Demux  Outputs=[1,1,1]
  Out1 : Outport  VectorParamsAs1DForOutWhenUnconnected=off
  wires:
  Demux/3 -> Bus Creator1/3  "Reactive power Q (var)"
  Demux/1 -> Bus Creator1/1  "Positive-sequence voltage V (pu)"
  Demux/2 -> Bus Creator1/2  "Active power P (W)"
  Bus Creator1/1 -> Out1/1
  In1/1 -> Demux/1

== system IEEE34_SPSload/SM_IEEE34/DL_858-834/Load B/model ==
  v : Inport
  PQ : Inport  Port=2
  Break Alg. Loop : Subsystem
  Complex to Magnitude-Angle : ComplexToMagnitudeAngle
  Complex to Real-Imag1 : ComplexToRealImag
  Constant : Constant
  Demux : Demux  Outputs=2
      settings: DisplayOption=none
  Divide : Product  Inputs=**
  IC1 : InitialCondition
  IC2 : InitialCondition
  Magnitude-Angle to Complex : MagnitudeAngleToComplex
  PLL : Subsystem  mask{freq=fnom}
      mask prompts: freq "Initial frequency (Hz)"
  Positive Sequence current : Subsystem
  RMS1 : spsRMSLib/RMS  TrueRMS=on  Freq=fnom  RMSInit=1  Ts=0
  Real-Imag to Complex : RealImagToComplex
  Real-Imag to Complex1 : RealImagToComplex
  Sum : Sum
  Trigonometric Function1 : Trigonometry
  V> pu : Gain  Gain=1/Vbase/sqrt(3)  SaturateOnIntegerOverflow=on  OutDataTypeStr=Inherit: Same as input  ParamDataTypeStr=Inherit: Same as input
  V> pu1 : Gain  Gain=sqrt(2)  SaturateOnIntegerOverflow=on  OutDataTypeStr=Inherit: Same as input  ParamDataTypeStr=Inherit: Same as input
  i : Outport  VectorParamsAs1DForOutWhenUnconnected=off
  m : Outport  Port=2  VectorParamsAs1DForOutWhenUnconnected=off
  wires:
  V> pu/1 -> PLL/1(v (pu)), V> pu1/1
  Real-Imag to Complex/1 -> Positive Sequence current/1(V1(pu))
  Positive Sequence current/1(I1(A)) -> Break Alg. Loop/1(In)
  PQ/1 -> Demux/1
  Demux/1 -> Real-Imag to Complex1/1
  Demux/2 -> Real-Imag to Complex1/2
  Real-Imag to Complex1/1 -> Positive Sequence current/2(S_ext)
  Positive Sequence current/2(VPQ) -> m/1
  v/1 -> IC2/1
  Complex to Real-Imag1/1 -> Real-Imag to Complex/1
  Complex to Real-Imag1/2 -> Real-Imag to Complex/2
  Magnitude-Angle to Complex/1 -> Complex to Real-Imag1/1
  Constant/1 -> PLL/2(freq (pu))
  PLL/1(alpha (rad)) -> Magnitude-Angle to Complex/2
  Complex to Magnitude-Angle/2 -> Sum/2
  PLL/2(wt) -> Sum/1
  Sum/1 -> Trigonometric Function1/1
  Trigonometric Function1/1 -> Divide/2
  Complex to Magnitude-Angle/1 -> Divide/1
  Divide/1 -> i/1
  Break Alg. Loop/1(Out) -> Complex to Magnitude-Angle/1
  RMS1/1 -> IC1/1
  IC1/1 -> Magnitude-Angle to Complex/1
  V> pu1/1 -> RMS1/1
  IC2/1 -> V> pu/1

== system IEEE34_SPSload/SM_IEEE34/DL_858-834/Load B1/Measurement list ==
  In1 : Inport
  Bus Creator1 : BusCreator  Inputs=3
  Demux : Demux  Outputs=[1,1,1]
  Out1 : Outport  VectorParamsAs1DForOutWhenUnconnected=off
  wires:
  Demux/3 -> Bus Creator1/3  "Reactive power Q (var)"
  Demux/1 -> Bus Creator1/1  "Positive-sequence voltage V (pu)"
  Demux/2 -> Bus Creator1/2  "Active power P (W)"
  Bus Creator1/1 -> Out1/1
  In1/1 -> Demux/1

== system IEEE34_SPSload/SM_IEEE34/DL_858-834/Load B1/model ==
  v : Inport
  PQ : Inport  Port=2
  Break Alg. Loop : Subsystem
  Complex to Magnitude-Angle : ComplexToMagnitudeAngle
  Complex to Real-Imag1 : ComplexToRealImag
  Constant : Constant
  Demux : Demux  Outputs=2
      settings: DisplayOption=none
  Divide : Product  Inputs=**
  IC1 : InitialCondition
  IC2 : InitialCondition
  Magnitude-Angle to Complex : MagnitudeAngleToComplex
  PLL : Subsystem  mask{freq=fnom}
      mask prompts: freq "Initial frequency (Hz)"
  Positive Sequence current : Subsystem
  RMS1 : spsRMSLib/RMS  TrueRMS=on  Freq=fnom  RMSInit=1  Ts=0
  Real-Imag to Complex : RealImagToComplex
  Real-Imag to Complex1 : RealImagToComplex
  Sum : Sum
  Trigonometric Function1 : Trigonometry
  V> pu : Gain  Gain=1/Vbase/sqrt(3)  SaturateOnIntegerOverflow=on  OutDataTypeStr=Inherit: Same as input  ParamDataTypeStr=Inherit: Same as input
  V> pu1 : Gain  Gain=sqrt(2)  SaturateOnIntegerOverflow=on  OutDataTypeStr=Inherit: Same as input  ParamDataTypeStr=Inherit: Same as input
  i : Outport  VectorParamsAs1DForOutWhenUnconnected=off
  m : Outport  Port=2  VectorParamsAs1DForOutWhenUnconnected=off
  wires:
  V> pu/1 -> PLL/1(v (pu)), V> pu1/1
  Real-Imag to Complex/1 -> Positive Sequence current/1(V1(pu))
  Positive Sequence current/1(I1(A)) -> Break Alg. Loop/1(In)
  PQ/1 -> Demux/1
  Demux/1 -> Real-Imag to Complex1/1
  Demux/2 -> Real-Imag to Complex1/2
  Real-Imag to Complex1/1 -> Positive Sequence current/2(S_ext)
  Positive Sequence current/2(VPQ) -> m/1
  v/1 -> IC2/1
  Complex to Real-Imag1/1 -> Real-Imag to Complex/1
  Complex to Real-Imag1/2 -> Real-Imag to Complex/2
  Magnitude-Angle to Complex/1 -> Complex to Real-Imag1/1
  Constant/1 -> PLL/2(freq (pu))
  PLL/1(alpha (rad)) -> Magnitude-Angle to Complex/2
  Complex to Magnitude-Angle/2 -> Sum/2
  PLL/2(wt) -> Sum/1
  Sum/1 -> Trigonometric Function1/1
  Trigonometric Function1/1 -> Divide/2
  Complex to Magnitude-Angle/1 -> Divide/1
  Divide/1 -> i/1
  Break Alg. Loop/1(Out) -> Complex to Magnitude-Angle/1
  RMS1/1 -> IC1/1
  IC1/1 -> Magnitude-Angle to Complex/1
  V> pu1/1 -> RMS1/1
  IC2/1 -> V> pu/1

== system IEEE34_SPSload/SM_IEEE34/DL_858-834/Load B2/Measurement list ==
  In1 : Inport
  Bus Creator1 : BusCreator  Inputs=3
  Demux : Demux  Outputs=[1,1,1]
  Out1 : Outport  VectorParamsAs1DForOutWhenUnconnected=off
  wires:
  Demux/3 -> Bus Creator1/3  "Reactive power Q (var)"
  Demux/1 -> Bus Creator1/1  "Positive-sequence voltage V (pu)"
  Demux/2 -> Bus Creator1/2  "Active power P (W)"
  Bus Creator1/1 -> Out1/1
  In1/1 -> Demux/1

== system IEEE34_SPSload/SM_IEEE34/DL_858-834/Load B2/model ==
  v : Inport
  PQ : Inport  Port=2
  Break Alg. Loop : Subsystem
  Complex to Magnitude-Angle : ComplexToMagnitudeAngle
  Complex to Real-Imag1 : ComplexToRealImag
  Constant : Constant
  Demux : Demux  Outputs=2
      settings: DisplayOption=none
  Divide : Product  Inputs=**
  IC1 : InitialCondition
  IC2 : InitialCondition
  Magnitude-Angle to Complex : MagnitudeAngleToComplex
  PLL : Subsystem  mask{freq=fnom}
      mask prompts: freq "Initial frequency (Hz)"
  Positive Sequence current : Subsystem
  RMS1 : spsRMSLib/RMS  TrueRMS=on  Freq=fnom  RMSInit=1  Ts=0
  Real-Imag to Complex : RealImagToComplex
  Real-Imag to Complex1 : RealImagToComplex
  Sum : Sum
  Trigonometric Function1 : Trigonometry
  V> pu : Gain  Gain=1/Vbase/sqrt(3)  SaturateOnIntegerOverflow=on  OutDataTypeStr=Inherit: Same as input  ParamDataTypeStr=Inherit: Same as input
  V> pu1 : Gain  Gain=sqrt(2)  SaturateOnIntegerOverflow=on  OutDataTypeStr=Inherit: Same as input  ParamDataTypeStr=Inherit: Same as input
  i : Outport  VectorParamsAs1DForOutWhenUnconnected=off
  m : Outport  Port=2  VectorParamsAs1DForOutWhenUnconnected=off
  wires:
  V> pu/1 -> PLL/1(v (pu)), V> pu1/1
  Real-Imag to Complex/1 -> Positive Sequence current/1(V1(pu))
  Positive Sequence current/1(I1(A)) -> Break Alg. Loop/1(In)
  PQ/1 -> Demux/1
  Demux/1 -> Real-Imag to Complex1/1
  Demux/2 -> Real-Imag to Complex1/2
  Real-Imag to Complex1/1 -> Positive Sequence current/2(S_ext)
  Positive Sequence current/2(VPQ) -> m/1
  v/1 -> IC2/1
  Complex to Real-Imag1/1 -> Real-Imag to Complex/1
  Complex to Real-Imag1/2 -> Real-Imag to Complex/2
  Magnitude-Angle to Complex/1 -> Complex to Real-Imag1/1
  Constant/1 -> PLL/2(freq (pu))
  PLL/1(alpha (rad)) -> Magnitude-Angle to Complex/2
  Complex to Magnitude-Angle/2 -> Sum/2
  PLL/2(wt) -> Sum/1
  Sum/1 -> Trigonometric Function1/1
  Trigonometric Function1/1 -> Divide/2
  Complex to Magnitude-Angle/1 -> Divide/1
  Divide/1 -> i/1
  Break Alg. Loop/1(Out) -> Complex to Magnitude-Angle/1
  RMS1/1 -> IC1/1
  IC1/1 -> Magnitude-Angle to Complex/1
  V> pu1/1 -> RMS1/1
  IC2/1 -> V> pu/1

== system IEEE34_SPSload/SM_IEEE34/DL_858-864/Load B/Measurement list ==
  In1 : Inport
  Bus Creator1 : BusCreator  Inputs=3
  Demux : Demux  Outputs=[1,1,1]
  Out1 : Outport  VectorParamsAs1DForOutWhenUnconnected=off
  wires:
  Demux/3 -> Bus Creator1/3  "Reactive power Q (var)"
  Demux/1 -> Bus Creator1/1  "Positive-sequence voltage V (pu)"
  Demux/2 -> Bus Creator1/2  "Active power P (W)"
  Bus Creator1/1 -> Out1/1
  In1/1 -> Demux/1

== system IEEE34_SPSload/SM_IEEE34/DL_858-864/Load B/model ==
  v : Inport
  PQ : Inport  Port=2
  Break Alg. Loop : Subsystem
  Complex to Magnitude-Angle : ComplexToMagnitudeAngle
  Complex to Real-Imag1 : ComplexToRealImag
  Constant : Constant
  Demux : Demux  Outputs=2
      settings: DisplayOption=none
  Divide : Product  Inputs=**
  IC1 : InitialCondition
  IC2 : InitialCondition
  Magnitude-Angle to Complex : MagnitudeAngleToComplex
  PLL : Subsystem  mask{freq=fnom}
      mask prompts: freq "Initial frequency (Hz)"
  Positive Sequence current : Subsystem
  RMS1 : spsRMSLib/RMS  TrueRMS=on  Freq=fnom  RMSInit=1  Ts=0
  Real-Imag to Complex : RealImagToComplex
  Real-Imag to Complex1 : RealImagToComplex
  Sum : Sum
  Trigonometric Function1 : Trigonometry
  V> pu : Gain  Gain=1/Vbase/sqrt(3)  SaturateOnIntegerOverflow=on  OutDataTypeStr=Inherit: Same as input  ParamDataTypeStr=Inherit: Same as input
  V> pu1 : Gain  Gain=sqrt(2)  SaturateOnIntegerOverflow=on  OutDataTypeStr=Inherit: Same as input  ParamDataTypeStr=Inherit: Same as input
  i : Outport  VectorParamsAs1DForOutWhenUnconnected=off
  m : Outport  Port=2  VectorParamsAs1DForOutWhenUnconnected=off
  wires:
  V> pu/1 -> PLL/1(v (pu)), V> pu1/1
  Real-Imag to Complex/1 -> Positive Sequence current/1(V1(pu))
  Positive Sequence current/1(I1(A)) -> Break Alg. Loop/1(In)
  PQ/1 -> Demux/1
  Demux/1 -> Real-Imag to Complex1/1
  Demux/2 -> Real-Imag to Complex1/2
  Real-Imag to Complex1/1 -> Positive Sequence current/2(S_ext)
  Positive Sequence current/2(VPQ) -> m/1
  v/1 -> IC2/1
  Complex to Real-Imag1/1 -> Real-Imag to Complex/1
  Complex to Real-Imag1/2 -> Real-Imag to Complex/2
  Magnitude-Angle to Complex/1 -> Complex to Real-Imag1/1
  Constant/1 -> PLL/2(freq (pu))
  PLL/1(alpha (rad)) -> Magnitude-Angle to Complex/2
  Complex to Magnitude-Angle/2 -> Sum/2
  PLL/2(wt) -> Sum/1
  Sum/1 -> Trigonometric Function1/1
  Trigonometric Function1/1 -> Divide/2
  Complex to Magnitude-Angle/1 -> Divide/1
  Divide/1 -> i/1
  Break Alg. Loop/1(Out) -> Complex to Magnitude-Angle/1
  RMS1/1 -> IC1/1
  IC1/1 -> Magnitude-Angle to Complex/1
  V> pu1/1 -> RMS1/1
  IC2/1 -> V> pu/1

== system IEEE34_SPSload/SM_IEEE34/DL_860-1/Load A/Measurement list ==
  In1 : Inport
  Bus Creator1 : BusCreator  Inputs=3
  Demux : Demux  Outputs=[1,1,1]
  Out1 : Outport  VectorParamsAs1DForOutWhenUnconnected=off
  wires:
  In1/1 -> Demux/1
  Bus Creator1/1 -> Out1/1
  Demux/2 -> Bus Creator1/2  "Active power P (W)"
  Demux/1 -> Bus Creator1/1  "Positive-sequence voltage V (pu)"
  Demux/3 -> Bus Creator1/3  "Reactive power Q (var)"

== system IEEE34_SPSload/SM_IEEE34/DL_860-1/Load A/model ==
  v : Inport
  PQ : Inport  Port=2
  Break Alg. Loop : Subsystem
  Complex to Magnitude-Angle : ComplexToMagnitudeAngle
  Complex to Real-Imag1 : ComplexToRealImag
  Constant : Constant
  Demux : Demux  Outputs=2
      settings: DisplayOption=none
  Divide : Product  Inputs=**
  IC1 : InitialCondition
  IC2 : InitialCondition
  Magnitude-Angle to Complex : MagnitudeAngleToComplex
  PLL : Subsystem  mask{freq=fnom}
      mask prompts: freq "Initial frequency (Hz)"
  Positive Sequence current : Subsystem
  RMS1 : spsRMSLib/RMS  TrueRMS=on  Freq=fnom  RMSInit=1  Ts=0
  Real-Imag to Complex : RealImagToComplex
  Real-Imag to Complex1 : RealImagToComplex
  Sum : Sum
  Trigonometric Function1 : Trigonometry
  V> pu : Gain  Gain=1/Vbase/sqrt(3)  SaturateOnIntegerOverflow=on  OutDataTypeStr=Inherit: Same as input  ParamDataTypeStr=Inherit: Same as input
  V> pu1 : Gain  Gain=sqrt(2)  SaturateOnIntegerOverflow=on  OutDataTypeStr=Inherit: Same as input  ParamDataTypeStr=Inherit: Same as input
  i : Outport  VectorParamsAs1DForOutWhenUnconnected=off
  m : Outport  Port=2  VectorParamsAs1DForOutWhenUnconnected=off
  wires:
  IC2/1 -> V> pu/1
  V> pu1/1 -> RMS1/1
  IC1/1 -> Magnitude-Angle to Complex/1
  RMS1/1 -> IC1/1
  Break Alg. Loop/1(Out) -> Complex to Magnitude-Angle/1
  Divide/1 -> i/1
  Complex to Magnitude-Angle/1 -> Divide/1
  Trigonometric Function1/1 -> Divide/2
  Sum/1 -> Trigonometric Function1/1
  PLL/2(wt) -> Sum/1
  Complex to Magnitude-Angle/2 -> Sum/2
  PLL/1(alpha (rad)) -> Magnitude-Angle to Complex/2
  Constant/1 -> PLL/2(freq (pu))
  Magnitude-Angle to Complex/1 -> Complex to Real-Imag1/1
  Complex to Real-Imag1/2 -> Real-Imag to Complex/2
  Complex to Real-Imag1/1 -> Real-Imag to Complex/1
  v/1 -> IC2/1
  Positive Sequence current/2(VPQ) -> m/1
  Real-Imag to Complex1/1 -> Positive Sequence current/2(S_ext)
  Demux/2 -> Real-Imag to Complex1/2
  Demux/1 -> Real-Imag to Complex1/1
  PQ/1 -> Demux/1
  Positive Sequence current/1(I1(A)) -> Break Alg. Loop/1(In)
  Real-Imag to Complex/1 -> Positive Sequence current/1(V1(pu))
  V> pu/1 -> V> pu1/1, PLL/1(v (pu))

== system IEEE34_SPSload/SM_IEEE34/DL_860-1/Load B/Measurement list ==
  In1 : Inport
  Bus Creator1 : BusCreator  Inputs=3
  Demux : Demux  Outputs=[1,1,1]
  Out1 : Outport  VectorParamsAs1DForOutWhenUnconnected=off
  wires:
  In1/1 -> Demux/1
  Bus Creator1/1 -> Out1/1
  Demux/2 -> Bus Creator1/2  "Active power P (W)"
  Demux/1 -> Bus Creator1/1  "Positive-sequence voltage V (pu)"
  Demux/3 -> Bus Creator1/3  "Reactive power Q (var)"

== system IEEE34_SPSload/SM_IEEE34/DL_860-1/Load B/model ==
  v : Inport
  PQ : Inport  Port=2
  Break Alg. Loop : Subsystem
  Complex to Magnitude-Angle : ComplexToMagnitudeAngle
  Complex to Real-Imag1 : ComplexToRealImag
  Constant : Constant
  Demux : Demux  Outputs=2
      settings: DisplayOption=none
  Divide : Product  Inputs=**
  IC1 : InitialCondition
  IC2 : InitialCondition
  Magnitude-Angle to Complex : MagnitudeAngleToComplex
  PLL : Subsystem  mask{freq=fnom}
      mask prompts: freq "Initial frequency (Hz)"
  Positive Sequence current : Subsystem
  RMS1 : spsRMSLib/RMS  TrueRMS=on  Freq=fnom  RMSInit=1  Ts=0
  Real-Imag to Complex : RealImagToComplex
  Real-Imag to Complex1 : RealImagToComplex
  Sum : Sum
  Trigonometric Function1 : Trigonometry
  V> pu : Gain  Gain=1/Vbase/sqrt(3)  SaturateOnIntegerOverflow=on  OutDataTypeStr=Inherit: Same as input  ParamDataTypeStr=Inherit: Same as input
  V> pu1 : Gain  Gain=sqrt(2)  SaturateOnIntegerOverflow=on  OutDataTypeStr=Inherit: Same as input  ParamDataTypeStr=Inherit: Same as input
  i : Outport  VectorParamsAs1DForOutWhenUnconnected=off
  m : Outport  Port=2  VectorParamsAs1DForOutWhenUnconnected=off
  wires:
  IC2/1 -> V> pu/1
  V> pu1/1 -> RMS1/1
  IC1/1 -> Magnitude-Angle to Complex/1
  RMS1/1 -> IC1/1
  Break Alg. Loop/1(Out) -> Complex to Magnitude-Angle/1
  Divide/1 -> i/1
  Complex to Magnitude-Angle/1 -> Divide/1
  Trigonometric Function1/1 -> Divide/2
  Sum/1 -> Trigonometric Function1/1
  PLL/2(wt) -> Sum/1
  Complex to Magnitude-Angle/2 -> Sum/2
  PLL/1(alpha (rad)) -> Magnitude-Angle to Complex/2
  Constant/1 -> PLL/2(freq (pu))
  Magnitude-Angle to Complex/1 -> Complex to Real-Imag1/1
  Complex to Real-Imag1/2 -> Real-Imag to Complex/2
  Complex to Real-Imag1/1 -> Real-Imag to Complex/1
  v/1 -> IC2/1
  Positive Sequence current/2(VPQ) -> m/1
  Real-Imag to Complex1/1 -> Positive Sequence current/2(S_ext)
  Demux/2 -> Real-Imag to Complex1/2
  Demux/1 -> Real-Imag to Complex1/1
  PQ/1 -> Demux/1
  Positive Sequence current/1(I1(A)) -> Break Alg. Loop/1(In)
  Real-Imag to Complex/1 -> Positive Sequence current/1(V1(pu))
  V> pu/1 -> V> pu1/1, PLL/1(v (pu))

== system IEEE34_SPSload/SM_IEEE34/DL_860-1/Load C/Measurement list ==
  In1 : Inport
  Bus Creator1 : BusCreator  Inputs=3
  Demux : Demux  Outputs=[1,1,1]
  Out1 : Outport  VectorParamsAs1DForOutWhenUnconnected=off
  wires:
  In1/1 -> Demux/1
  Bus Creator1/1 -> Out1/1
  Demux/2 -> Bus Creator1/2  "Active power P (W)"
  Demux/1 -> Bus Creator1/1  "Positive-sequence voltage V (pu)"
  Demux/3 -> Bus Creator1/3  "Reactive power Q (var)"
